simulink model "DoAero"  (Simulink 8.5)
settings: Solver=ode3  StartTime=0.0  StopTime=10  FixedStep=0.01  RelTol=1e-3
settings Model: Creator=abdelrazzak.merheb  LastModifiedBy=flying
settings DataIOCC: ExternalInput=getinputstruct(op_trim1)  InitialState=getstatestruct(op_trim1)
settings OptimizationCC: InlineParams=on  BufferReuse=off
settings DebuggingCC: SolverPrmCheckMsg=warning  FcnCallInpInsideContextMsg=UseLocalSettings  InitInArrayFormatMsg=none

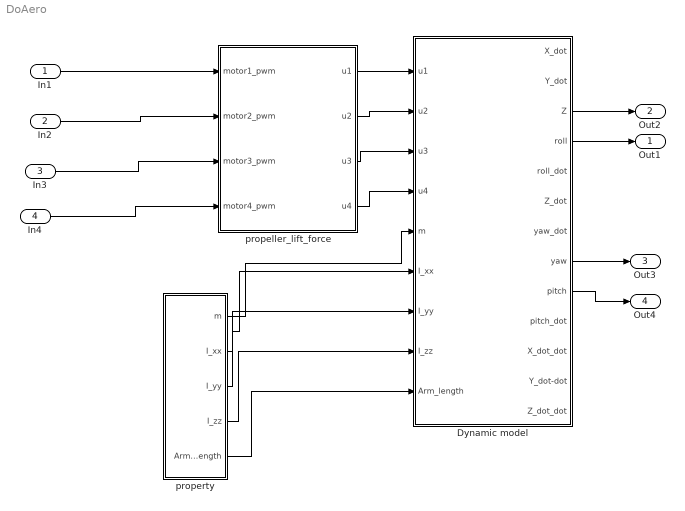
== system DoAero ==
  In1 : Inport
  In2 : Inport  Port=2
  In3 : Inport  Port=3
  In4 : Inport  Port=4
  Dynamic model : Subsystem
  propeller_lift_force : MATLAB Function  TreatAsAtomicUnit=on
  "property " : Subsystem
  Out1 : Outport
  Out2 : Outport  Port=2
  Out3 : Outport  Port=3
  Out4 : Outport  Port=4
  wires:
  "property "/5("Arm_length ") -> Dynamic model/9(Arm_length)
  "property "/4(I_zz) -> Dynamic model/8(I_zz)
  "property "/3(I_yy) -> Dynamic model/7(I_yy)
  "property "/2(I_xx) -> Dynamic model/6(I_xx)
  "property "/1(m) -> Dynamic model/5(m)
  propeller_lift_force/2(u2) -> Dynamic model/2(u2)
  propeller_lift_force/3(u3) -> Dynamic model/3(u3)
  propeller_lift_force/1(u1) -> Dynamic model/1(u1)
  propeller_lift_force/4(u4) -> Dynamic model/4(u4)
  In4/1 -> propeller_lift_force/4(motor4_pwm)
  In3/1 -> propeller_lift_force/3(motor3_pwm)
  In2/1 -> propeller_lift_force/2(motor2_pwm)
  In1/1 -> propeller_lift_force/1(motor1_pwm)
  Dynamic model/4(roll) -> Out1/1
  Dynamic model/3(Z) -> Out2/1
  Dynamic model/8(yaw) -> Out3/1
  Dynamic model/9(pitch) -> Out4/1

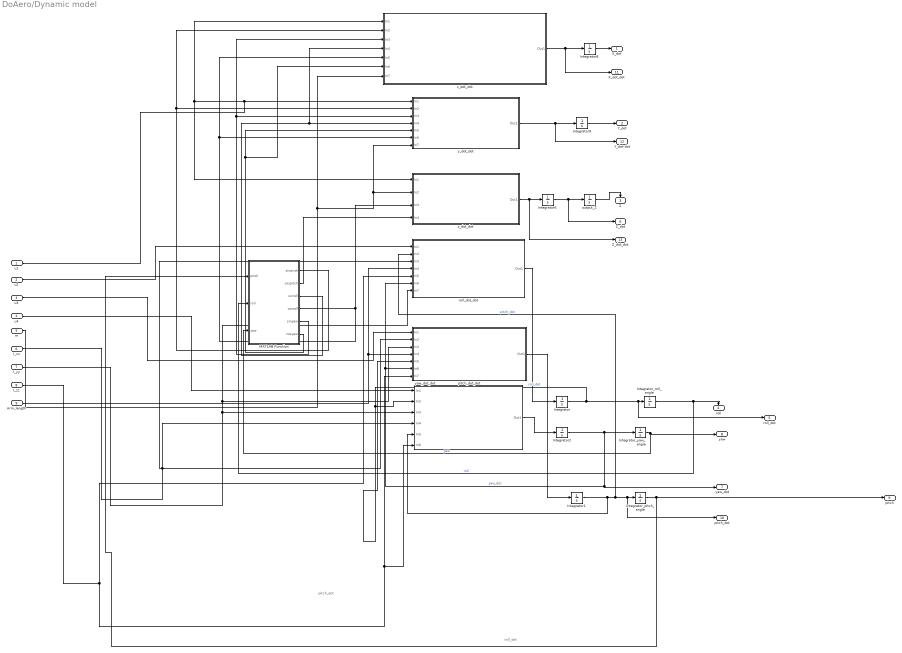
== system DoAero/Dynamic model ==
  note: pitch_dot
  note: roll_dot
  u1 : Inport
  u2 : Inport  Port=2
  u3 : Inport  Port=3
  u4 : Inport  Port=4
  m : Inport  Port=5
  I_xx : Inport  Port=6
  I_yy : Inport  Port=7
  I_zz : Inport  Port=8
  Arm_length : Inport  Port=9
  Integrator{,1..2,6,8..9} (6 alike) : Integrator
  Integrator_pitch_angle : Integrator
  Integrator_roll_angle : Integrator
  Integrator_yaw_angle : Integrator
  MATLAB Function : MATLAB Function  TreatAsAtomicUnit=on
  output_Z : Integrator
  pitch_dot_dot : Subsystem
  roll_dot_dot : Subsystem
  x_dot_dot : Subsystem
  y_dot_dot : Subsystem
  yaw_dot_dot : Subsystem
  z_dot_dot : Subsystem
  "X_dot " : Outport
  Y_dot : Outport  Port=2
  Z : Outport  Port=3
  roll : Outport  Port=4
  roll_dot : Outport  Port=5
  Z_dot : Outport  Port=6
  yaw_dot : Outport  Port=7
  yaw : Outport  Port=8
  pitch : Outport  Port=9
  pitch_dot : Outport  Port=10
  X_dot_dot : Outport  Port=11
  Y_dot-dot : Outport  Port=12
  Z_dot_dot : Outport  Port=13
  wires:
  x_dot_dot/1(Out1) -> X_dot_dot/1, Integrator8/1
  Integrator6/1 -> output_Z/1, Z_dot/1
  u4/1 -> yaw_dot_dot/1(In1)
  MATLAB Function/6(cosyaw) -> x_dot_dot/6(In6), y_dot_dot/5(In5)
  MATLAB Function/3(sinroll) -> x_dot_dot/4(In4), y_dot_dot/4(In4)
  MATLAB Function/4(cosroll) -> x_dot_dot/5(In5), y_dot_dot/6(In6), z_dot_dot/3(In3)
  MATLAB Function/1(sinpitch) -> x_dot_dot/2(In2), y_dot_dot/2(In2)
  m/1 -> x_dot_dot/7(In7), z_dot_dot/2(In2), y_dot_dot/7(In7)
  MATLAB Function/5(sinyaw) -> x_dot_dot/3(In3), y_dot_dot/3(In3)
  u1/1 -> y_dot_dot/1(In1), x_dot_dot/1(In1), z_dot_dot/1(In1)
  I_xx/1 -> yaw_dot_dot/4(In4), roll_dot_dot/3(In3), pitch_dot_dot/2(In2)
  I_yy/1 -> yaw_dot_dot/3(In3), roll_dot_dot/7(In7), pitch_dot_dot/3(In3)
  I_zz/1 -> roll_dot_dot/5(In5), yaw_dot_dot/6(In6), pitch_dot_dot/7(In7)
  Integrator_roll_angle/1 -> roll/1, MATLAB Function/2(roll)  "roll"
  Integrator1/1 -> yaw_dot_dot/5(In5), roll_dot_dot/2(In2), pitch_dot/1, Integrator_pitch_angle/1  "pitch_dot"
  Integrator2/1 -> roll_dot_dot/6(In6), pitch_dot_dot/6(In6), yaw_dot/1, Integrator_yaw_angle/1  "yaw_dot"
  Integrator/1 -> pitch_dot_dot/5(In5), yaw_dot_dot/2(In2), roll_dot/1, Integrator_roll_angle/1  "roll_dot"
  Integrator8/1 -> "X_dot "/1
  Integrator9/1 -> Y_dot/1
  Integrator_yaw_angle/1 -> MATLAB Function/3(yaw), yaw/1  "yaw"
  z_dot_dot/1(Out1) -> Z_dot_dot/1, Integrator6/1
  roll_dot_dot/1(Out1) -> Integrator/1
  pitch_dot_dot/1(Out1) -> Integrator1/1
  MATLAB Function/2(cospitch) -> z_dot_dot/4(In4)
  u2/1 -> roll_dot_dot/1(In1)
  Arm_length/1 -> roll_dot_dot/4(In4), pitch_dot_dot/4(In4)
  u3/1 -> pitch_dot_dot/1(In1)
  y_dot_dot/1(Out1) -> Y_dot-dot/1, Integrator9/1
  Integrator_pitch_angle/1 -> pitch/1, MATLAB Function/1(pitch)
  output_Z/1 -> Z/1
  yaw_dot_dot/1(Out1) -> Integrator2/1

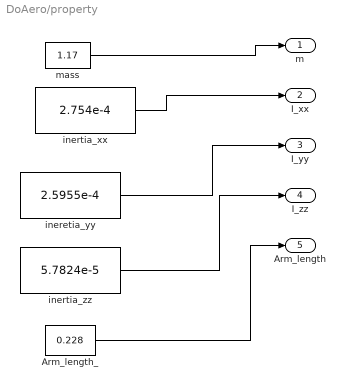
== system DoAero/property  ==
  Arm_length_ : Constant  Value=0.228
  ineretia_yy : Constant  Value=2.5955e-4
  inertia_xx : Constant  Value=2.754e-4
  inertia_zz : Constant  Value=5.7824e-5
  mass : Constant  Value=1.17
  m : Outport
  I_xx : Outport  Port=2
  I_yy : Outport  Port=3
  I_zz : Outport  Port=4
  "Arm_length " : Outport  Port=5
  wires:
  inertia_zz/1 -> I_zz/1
  Arm_length_/1 -> "Arm_length "/1
  ineretia_yy/1 -> I_yy/1
  mass/1 -> m/1
  inertia_xx/1 -> I_xx/1

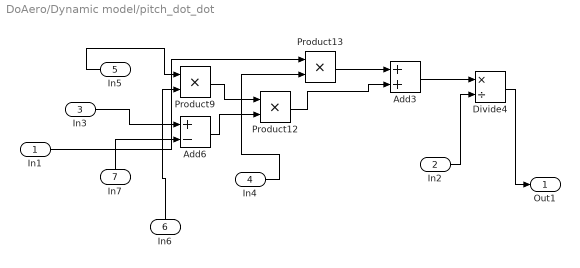
== system DoAero/Dynamic model/pitch_dot_dot ==
  In1 : Inport
  In2 : Inport  Port=2
  In3 : Inport  Port=3
  In4 : Inport  Port=4
  In5 : Inport  Port=5
  In6 : Inport  Port=6
  In7 : Inport  Port=7
  Add3 : Sum
  Add6 : Sum  Inputs=+-
  Divide4 : Product  Inputs=*/
  Product12 : Product
  Product13 : Product
  Product9 : Product
  Out1 : Outport
  wires:
  Product12/1 -> Add3/2
  Product13/1 -> Add3/1
  In1/1 -> Product13/1
  Add6/1 -> Product12/2
  Add3/1 -> Divide4/1
  Product9/1 -> Product12/1
  In4/1 -> Product13/2
  In6/1 -> Product9/2
  In7/1 -> Add6/2
  In3/1 -> Add6/1
  In2/1 -> Divide4/2
  In5/1 -> Product9/1
  Divide4/1 -> Out1/1

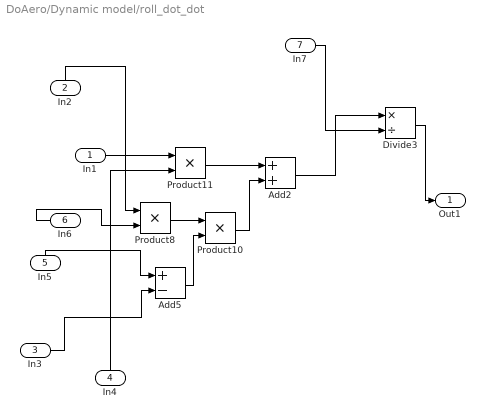
== system DoAero/Dynamic model/roll_dot_dot ==
  In1 : Inport
  In2 : Inport  Port=2
  In3 : Inport  Port=3
  In4 : Inport  Port=4
  In5 : Inport  Port=5
  In6 : Inport  Port=6
  In7 : Inport  Port=7
  Add2 : Sum
  Add5 : Sum  Inputs=+-
  Divide3 : Product  Inputs=*/
  Product10 : Product
  Product11 : Product
  Product8 : Product
  Out1 : Outport
  wires:
  Product11/1 -> Add2/1
  Add5/1 -> Product10/2
  In1/1 -> Product11/1
  Add2/1 -> Divide3/1
  Product8/1 -> Product10/1
  Product10/1 -> Add2/2
  Divide3/1 -> Out1/1
  In5/1 -> Add5/1
  In3/1 -> Add5/2
  In2/1 -> Product8/1
  In7/1 -> Divide3/2
  In4/1 -> Product11/2
  In6/1 -> Product8/2

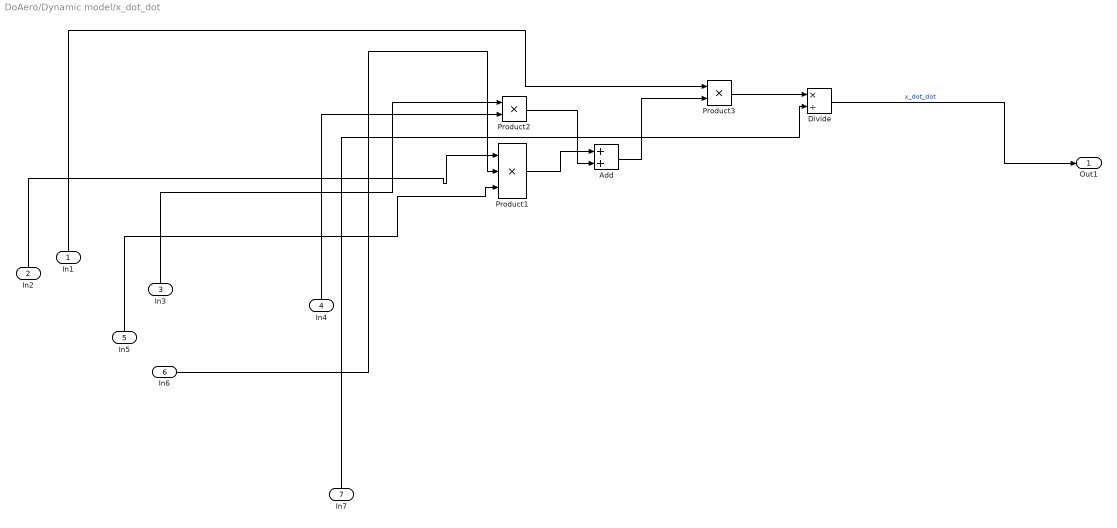
== system DoAero/Dynamic model/x_dot_dot ==
  In1 : Inport
  In2 : Inport  Port=2
  In3 : Inport  Port=3
  In4 : Inport  Port=4
  In5 : Inport  Port=5
  In6 : Inport  Port=6
  In7 : Inport  Port=7
  Add : Sum
  Divide : Product  Inputs=*/
  Product1 : Product  Inputs=3
  Product2 : Product
  Product3 : Product
  Out1 : Outport
  wires:
  In1/1 -> Product3/1
  In6/1 -> Product1/2
  In7/1 -> Divide/2
  In4/1 -> Product2/2
  In3/1 -> Product2/1
  In5/1 -> Product1/3
  In2/1 -> Product1/1
  Divide/1 -> Out1/1  "x_dot_dot"
  Product2/1 -> Add/2
  Product1/1 -> Add/1
  Product3/1 -> Divide/1
  Add/1 -> Product3/2

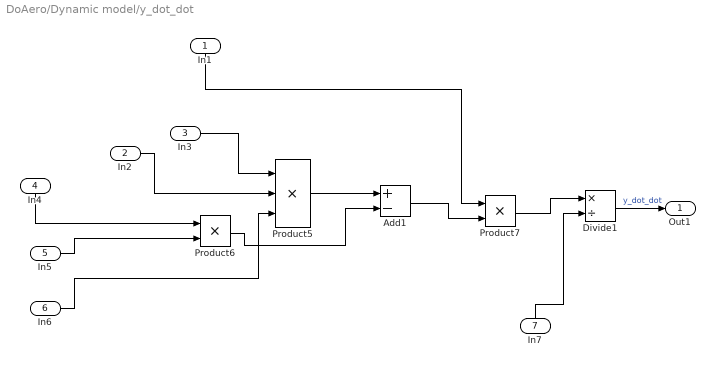
== system DoAero/Dynamic model/y_dot_dot ==
  In1 : Inport
  In2 : Inport  Port=2
  In3 : Inport  Port=3
  In4 : Inport  Port=4
  In5 : Inport  Port=5
  In6 : Inport  Port=6
  In7 : Inport  Port=7
  Add1 : Sum  Inputs=+-
  Divide1 : Product  Inputs=*/
  Product5 : Product  Inputs=3
  Product6 : Product
  Product7 : Product
  Out1 : Outport
  wires:
  In1/1 -> Product7/1
  In2/1 -> Product5/2
  In5/1 -> Product6/2
  In7/1 -> Divide1/2
  In6/1 -> Product5/3
  In3/1 -> Product5/1
  In4/1 -> Product6/1
  Product5/1 -> Add1/1
  Add1/1 -> Product7/2
  Product6/1 -> Add1/2
  Divide1/1 -> Out1/1  "y_dot_dot"
  Product7/1 -> Divide1/1

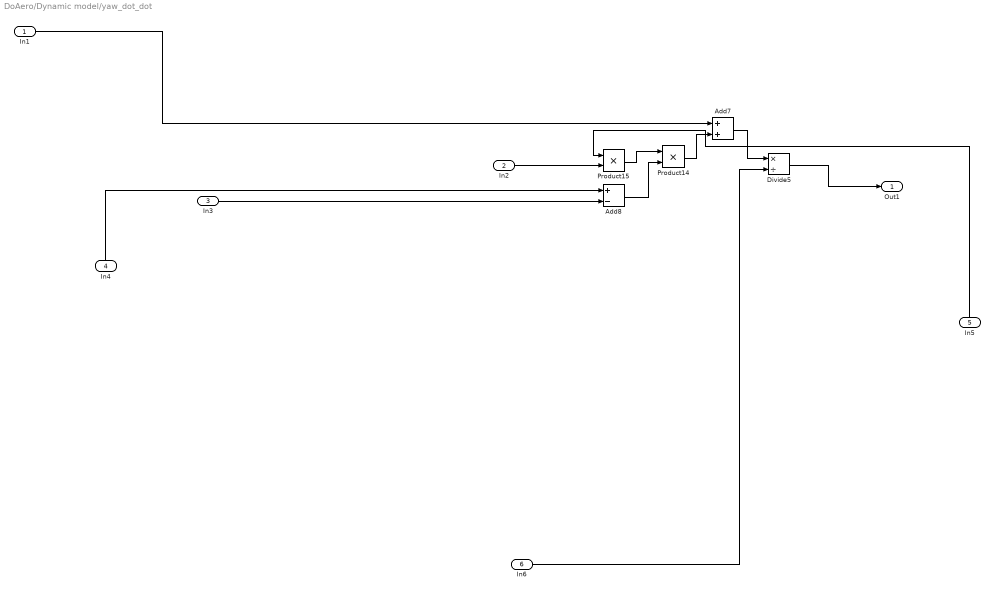
== system DoAero/Dynamic model/yaw_dot_dot ==
  In1 : Inport
  In2 : Inport  Port=2
  In3 : Inport  Port=3
  In4 : Inport  Port=4
  In5 : Inport  Port=5
  In6 : Inport  Port=6
  Add7 : Sum
  Add8 : Sum  Inputs=+-
  Divide5 : Product  Inputs=*/
  Product14 : Product
  Product15 : Product
  Out1 : Outport
  wires:
  In4/1 -> Add8/1
  In6/1 -> Divide5/2
  In2/1 -> Product15/2
  In3/1 -> Add8/2
  In5/1 -> Product15/1
  Product14/1 -> Add7/2
  Add8/1 -> Product14/2
  Product15/1 -> Product14/1
  In1/1 -> Add7/1
  Add7/1 -> Divide5/1
  Divide5/1 -> Out1/1

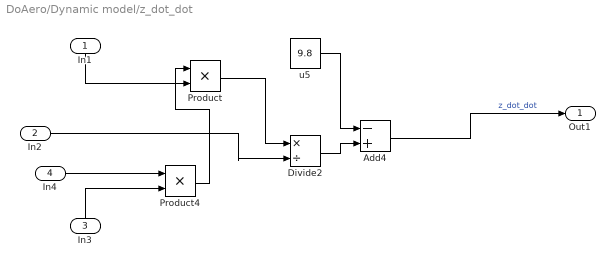
== system DoAero/Dynamic model/z_dot_dot ==
  In1 : Inport
  In2 : Inport  Port=2
  In3 : Inport  Port=3
  In4 : Inport  Port=4
  Add4 : Sum  Inputs=-+
  Divide2 : Product  Inputs=*/
  Product : Product
  Product4 : Product
  u5 : Constant  Value=9.8
  Out1 : Outport
  wires:
  In3/1 -> Product4/2
  In2/1 -> Divide2/2
  In1/1 -> Product/2
  Divide2/1 -> Add4/2
  Product4/1 -> Product/1
  In4/1 -> Product4/1
  u5/1 -> Add4/1
  Product/1 -> Divide2/1
  Add4/1 -> Out1/1  "z_dot_dot"

== matlab function propeller_lift_force ==
  data: motor1_pwm input double; u1 output double; motor2_pwm input double; motor3_pwm input double; motor4_pwm input double; u2 output double; u3 output double; u4 output double
function [u1,u2,u3,u4] = fcn(motor1_pwm,motor2_pwm,motor3_pwm,motor4_pwm)

n1=(motor1_pwm-1050)*7.054+900;
n2=(motor2_pwm-1050)*7.054+900;
n3=(motor3_pwm-1050)*7.054+900;
n4=(motor4_pwm-1050)*7.054+900;


F1=1.0384e-7*n1^2;
F2=1.0384e-7*n2^2;
F3=1.0384e-7*n3^2;
F4=1.0384e-7*n4^2;

u1=F1+F2+F3+F4;
u2=F4-F2;
u3=F3-F1;
u4=F2+F4-F1-F3;

== matlab function Dynamic model/MATLAB Function ==
  data: pitch input double; sinpitch output double; roll input double; yaw input double; cospitch output double; sinroll output double; cosroll output double; sinyaw output double; cosyaw output double
function [sinpitch,cospitch,sinroll,cosroll,sinyaw,cosyaw]= fcn(pitch,roll,yaw)
sinpitch=sin(pitch);
cospitch=cos(pitch);
sinroll=sin(roll);
cosroll=cos(roll);
sinyaw=sin(yaw);
cosyaw=cos(yaw);
